simulink model "sf_multioutput"  (R2017b)
settings: Solver=FixedStepDiscrete  StartTime=0.0  StopTime=10.0  FixedStep=1  RelTol=1e-3  EnableMultiTasking=on
settings Model: Creator=The MathWorks, Inc.  LastModifiedBy=The MathWorks, Inc.
settings DataIOCC: LimitDataPoints=on  SaveFormat=Array
settings OptimizationCC: ExpressionDepthLimit=2147483647  EfficientMapNaN2IntZero=off  LifeSpan=inf
settings DebuggingCC: UnderspecifiedInitializationDetection=Classic  MergeDetectMultiDrivingBlocksExec=none  SolverPrmCheckMsg=warning  FcnCallInpInsideContextMsg=warning  StateNameClashWarn=warning  StrictBusMsg=Warning  SFUnexpectedBacktrackingDiag=warning  SFNoUnconditionalDefaultTransitionDiag=warning  SFExecutionAtInitializationDiag=none
settings HardwareCC: ProdBitPerPointer=32  ProdBitPerSizeT=32  ProdBitPerPtrDiffT=32  ProdLargestAtomicFloat=None  ProdIntDivRoundTo=Undefined  ProdEndianess=Unspecified  ProdWordSize=32  ProdHWDeviceType=32-bit Generic
settings ModelReferenceCC: PropagateSignalLabelsOutOfModel=off
settings SFSimCC: SimParseCustomCode=off
settings CodeAppCC: StateflowObjectComments=on
settings GRTTargetCC: TargetLangStandard=C89/C90 (ANSI)  GeneratePreprocessorConditionals=Disable all  CombineOutputUpdateFcns=off  GRTInterface=on
settings ConfigComp: CovMetricSettings=dw  CovHtmlReporting=on  CovSaveCumulativeToWorkspaceVar=on  CovSaveSingleToWorkspaceVar=on  CovExternalEMLEnable=off  CovSFcnEnable=off

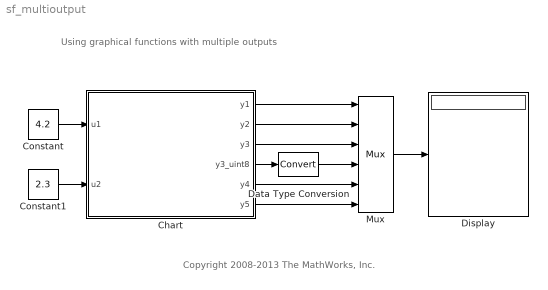
== system sf_multioutput ==
  note: Using graphical functions with multiple outputs
  note: Copyright 2008-2013 The MathWorks, Inc.
  Chart : Stateflow chart  TreatAsAtomicUnit=on
  Constant : Constant  Value=4.2
  Constant1 : Constant  Value=2.3
  Data Type Conversion : DataTypeConversion
  Display : Display
  Mux : Mux  Inputs=6
  wires:
  Chart/1(y1) -> Mux/1
  Chart/2(y2) -> Mux/2
  Chart/3(y3) -> Mux/3
  Chart/4(y3_uint8) -> Data Type Conversion/1
  Chart/5(y4) -> Mux/5
  Chart/6(y5) -> Mux/6
  Mux/1 -> Display/1
  Constant/1 -> Chart/1(u1)
  Constant1/1 -> Chart/2(u2)
  Data Type Conversion/1 -> Mux/4

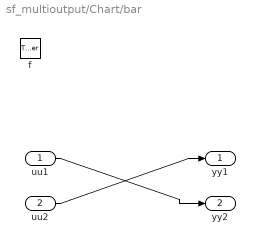
== system sf_multioutput/Chart/bar ==
  uu1 : Inport
  uu2 : Inport  Port=2
  f : TriggerPort  TriggerType=function-call  VariantControl=(inherit)
      settings: CopyFcn=Stateflow.SLINSF.SimulinkMan.removeBlockPreDeleteFcn  PreDeleteFcn=Stateflow.SLINSF.SimulinkMan.unsafePredeleteFcn
  yy1 : Outport
  yy2 : Outport  Port=2
  wires:
  uu1/1 -> yy2/1
  uu2/1 -> yy1/1

== stateflow chart sf_multioutput/Chart ==
  state [yy1,yy2] = bar(uu1,uu2) [function]
  state [yy1,yy2] = foo(uu1,uu2) [function]
    (default) -> (junction 9) : {yy1 = uu1 + uu2;
        |  yy2 = uu1 - uu2;}
  (default) -> (junction 2) : {
      | // Use standard MATLAB syntax to call multi output functions.
      | [y1,y2] = foo(u1,u2);
      |
      | // Multi output functions can be called with less than the full
      | // number of output arguments. In this case, the rest of the outputs
      | // are silently discarded. Used in an expression context, only the
      | // first output argument is used.
      | y3 = foo(u1,u2) * 3;
      |
      | // Outputs can be of a different type than the formal output types. In
      | // this case, the formal output is cast to the type of the assigned variable.
      | y3_uint8 = foo(u1,u2);
      |
      | // You can also use multiple outputs with MATLAB functions, Truth
      | // table and Simulink functions. Here we show a Simulink function.
      | [y4,y5] = bar(u1,u2);
      | }
  data: uu1 function_input; uu2 function_input; yy1 function_output; yy2 function_output; uu1 function_input double; uu2 function_input double; yy1 function_output double; yy2 function_output double; u1 input double; u2 input double; y1 output double; y2 output double; y3 output double; y3_uint8 output uint8; y4 output double; y5 output double
